simulink model "wurfparabel"  (R2014b)
settings: Solver=ode45  StartTime=0.0  StopTime=30.0  RelTol=1e-3
libraries: simulink x1
settings Model: Creator=sigurd  LastModifiedBy=sigurd

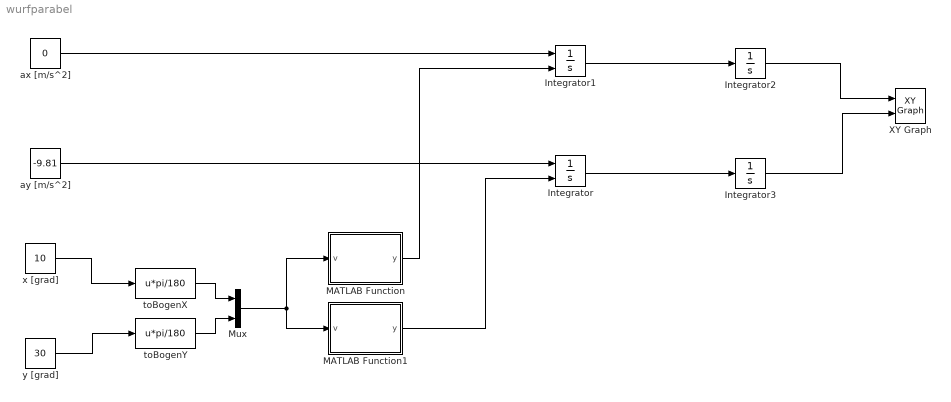
== system wurfparabel ==
  Integrator : Integrator  InitialConditionSource=external
  Integrator1 : Integrator  InitialConditionSource=external
  Integrator2 : Integrator
  Integrator3 : Integrator
  MATLAB Function : MATLAB Function  TreatAsAtomicUnit=on
  MATLAB Function1 : MATLAB Function  TreatAsAtomicUnit=on
  Mux : Mux  Inputs=2
  XY Graph : simulink/Sinks/XY Graph  xmin=-1  xmax=15  ymin=-1  ymax=5  st=-1
  ax [m/s^2] : Constant  Value=0
  ay [m/s^2] : Constant  Value=-9.81
  "toBogenX " : Fcn  Expr=u*pi/180
  toBogenY : Fcn  Expr=u*pi/180
  x [grad] : Constant  Value=10
  y [grad] : Constant  Value=30
  wires:
  x [grad]/1 -> "toBogenX "/1
  y [grad]/1 -> toBogenY/1
  Mux/1 -> MATLAB Function/1(v), MATLAB Function1/1(v)
  ax [m/s^2]/1 -> Integrator1/1
  ay [m/s^2]/1 -> Integrator/1
  Integrator/1 -> Integrator3/1
  Integrator1/1 -> Integrator2/1
  Integrator2/1 -> XY Graph/1
  Integrator3/1 -> XY Graph/2
  MATLAB Function/1(y) -> Integrator1/2
  MATLAB Function1/1(y) -> Integrator/2
  "toBogenX "/1 -> Mux/1
  toBogenY/1 -> Mux/2

== matlab function wurfparabel/MATLAB Function1 ==
  data: v input; y output
function y = fcn(v)
%#codegen

y =v(1)*sin(v(2));

== matlab function wurfparabel/MATLAB Function ==
  data: v input; y output
function y = fcn(v)
y = v(2)*cos(v(1));
